simulink model "MZI_3x3"  (R2019b)
settings: Solver=ode4  StartTime=0.0  StopTime=5  FixedStep=0.0001  RelTol=1e-3
values from neighbouring files (symbols this model uses):
  B = 2*pi/lambda    [Standing_wave_reflection_coef.m]
  C = 0.0043427    [accelerometer_estimated_sensitivity.m]
libraries: simulink x1
settings Model: Creator=Stinky  LastModifiedBy=Stinky

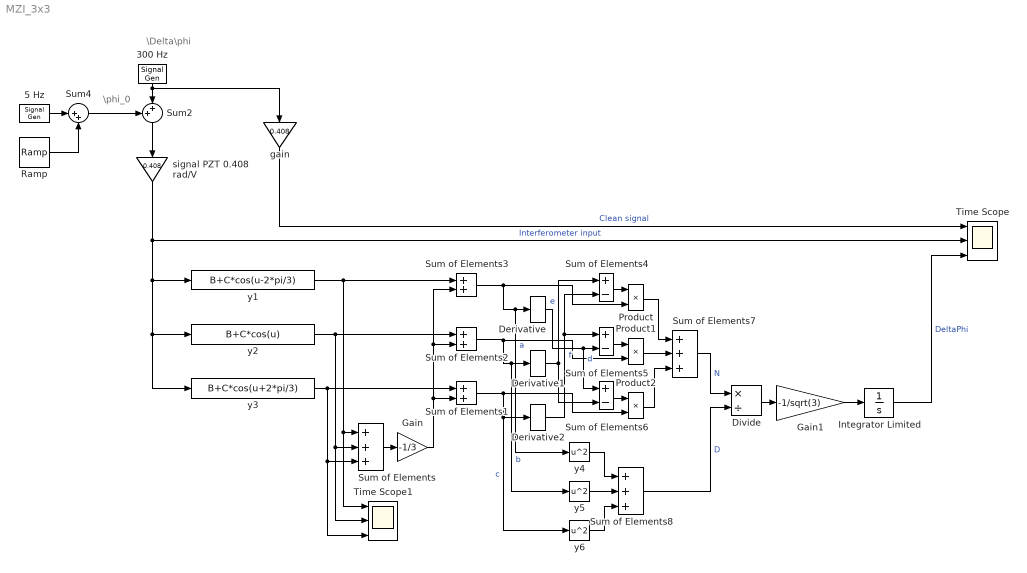
== system MZI_3x3 ==
  note: \phi_0
  note: \Delta\phi
  " 5 Hz" : SignalGenerator  Amplitude=2  Frequency=5
  "300 Hz " : SignalGenerator  Frequency=300
  Derivative : Derivative
  Derivative1 : Derivative
  Derivative2 : Derivative
  Divide : Product  Inputs=*/
  Gain : Gain  Gain=-1/3
  Gain1 : Gain  Gain=-1/sqrt(3)
  Integrator Limited : Integrator  LimitOutput=on  UpperSaturationLimit=1  LowerSaturationLimit=0
  Product : Product
  Product1 : Product
  Product2 : Product
  Ramp : simulink/Sources/Ramp  slope=50  start=0  InitialOutput=0
  Sum of Elements : Sum  Inputs=+++
  Sum of Elements1 : Sum
  Sum of Elements2 : Sum
  Sum of Elements3 : Sum
  Sum of Elements4 : Sum  Inputs=+-
  Sum of Elements5 : Sum  Inputs=+-
  Sum of Elements6 : Sum  Inputs=+-
  Sum of Elements7 : Sum  Inputs=+++
  Sum of Elements8 : Sum  Inputs=+++
  Sum2 : Sum  Inputs=++|
  Sum4 : Sum  Inputs=|++
  Time Scope : Scope  NumInputPorts=3
  Time Scope1 : Scope  NumInputPorts=3
  gain : Gain  Gain=0.408
  signal PZT 0.408 rad/V : Gain  Gain=0.408
  y1 : Fcn  Expr=B+C*cos(u-2*pi/3)
  y2 : Fcn  Expr=B+C*cos(u)
  y3 : Fcn  Expr=B+C*cos(u+2*pi/3)
  y4 : Fcn  Expr=u^2
  y5 : Fcn  Expr=u^2
  y6 : Fcn  Expr=u^2
  wires:
  Ramp/1 -> Sum4/2
  gain/1 -> Time Scope/1  "Clean signal"
  " 5 Hz"/1 -> Sum4/1
  signal PZT 0.408 rad/V/1 -> y3/1, y2/1, y1/1, Time Scope/2  "Interferometer input"
  Sum4/1 -> Sum2/1
  "300 Hz "/1 -> Sum2/2, gain/1
  Sum2/1 -> signal PZT 0.408 rad/V/1
  y1/1 -> Sum of Elements3/1, Sum of Elements/1, Time Scope1/1
  y2/1 -> Sum of Elements2/1, Sum of Elements/2, Time Scope1/2
  y3/1 -> Sum of Elements1/1, Sum of Elements/3, Time Scope1/3
  Sum of Elements/1 -> Gain/1
  Gain/1 -> Sum of Elements1/2, Sum of Elements2/2, Sum of Elements3/2
  Sum of Elements3/1 -> Product/2, y4/1, Derivative/1  "a"
  Sum of Elements2/1 -> Product1/2, y5/1, Derivative1/1  "b"
  Sum of Elements1/1 -> Product2/2, y6/1, Derivative2/1  "c"
  Sum of Elements4/1 -> Product/1
  Sum of Elements5/1 -> Product1/1
  Sum of Elements6/1 -> Product2/1
  Derivative/1 -> Sum of Elements6/1, Sum of Elements5/2  "d"
  Derivative1/1 -> Sum of Elements4/1, Sum of Elements6/2  "e"
  Derivative2/1 -> Sum of Elements5/1, Sum of Elements4/2  "f"
  Product1/1 -> Sum of Elements7/2
  Product/1 -> Sum of Elements7/1
  Product2/1 -> Sum of Elements7/3
  y5/1 -> Sum of Elements8/2
  y4/1 -> Sum of Elements8/1
  y6/1 -> Sum of Elements8/3
  Sum of Elements7/1 -> Divide/1  "N"
  Sum of Elements8/1 -> Divide/2  "D"
  Divide/1 -> Gain1/1
  Gain1/1 -> Integrator Limited/1
  Integrator Limited/1 -> Time Scope/3  "DeltaPhi"
